simulink model "Q2"  (R2023a)
settings: Solver=VariableStepAuto  StartTime=0.0  StopTime=20  RelTol=1e-3
settings Model: Creator=DELL  LastModifiedBy=DELL

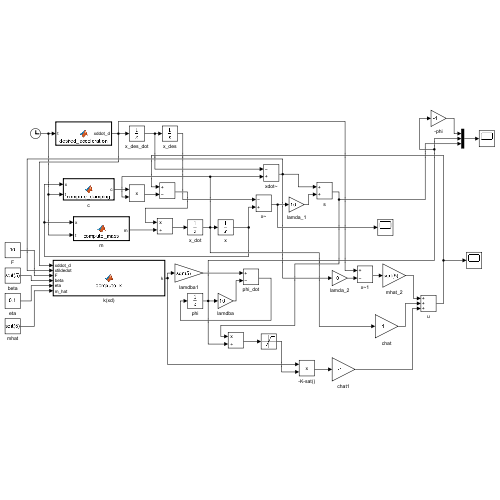
[thumbnail: Simulink's stored preview of the top-level diagram]
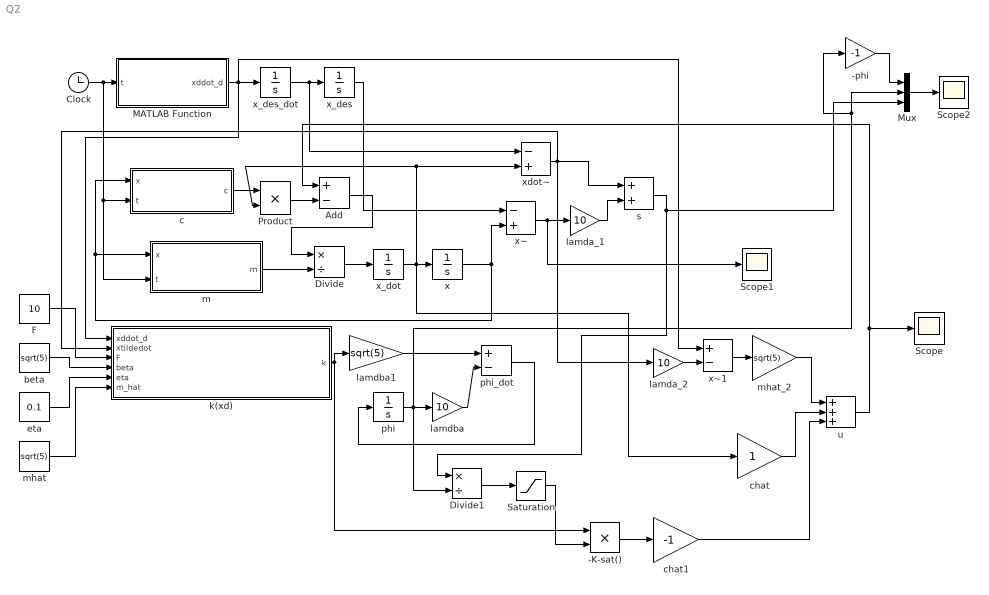
== system Q2 ==
  -K-sat() : Product  Inputs=**
  -phi : Gain  Gain=-1
  Add : Sum  Inputs=+-
  Clock : Clock
  Divide : Product  Inputs=*/
  Divide1 : Product  Inputs=*/
  F : Constant  Value=10
  MATLAB Function : MATLAB Function  TreatAsAtomicUnit=on
  Mux : Mux  Inputs=3
  Product : Product
  Saturation : Saturate  UpperLimit=1  LowerLimit=-1
  Scope : Scope
  Scope1 : Scope
  Scope2 : Scope
  beta : Constant  Value=sqrt(5)
  c : MATLAB Function  TreatAsAtomicUnit=on
  chat : Gain
  chat1 : Gain  Gain=-1
  eta : Constant  Value=0.1
  k(xd) : MATLAB Function  TreatAsAtomicUnit=on
  lamda_1 : Gain  Gain=10
  lamda_2 : Gain  Gain=10
  lamdba : Gain  Gain=10
  lamdba1 : Gain  Gain=sqrt(5)
  m : MATLAB Function  TreatAsAtomicUnit=on
  mhat : Constant  Value=sqrt(5)
  mhat_2 : Gain  Gain=sqrt(5)
  phi : Integrator  InitialCondition=0.01
  phi_dot : Sum  Inputs=+-
  s : Sum
  u : Sum  Inputs=+++
  x : Integrator
  x_des : Integrator
  x_des_dot : Integrator
  x_dot : Integrator
  xdot~ : Sum  Inputs=-+
  x~ : Sum  Inputs=-+
  x~1 : Sum  Inputs=+-
  wires:
  x_des_dot/1 -> xdot~/1, x_des/1
  Clock/1 -> c/2(t), m/2(t), MATLAB Function/1(t)
  MATLAB Function/1(xddot_d) -> x~1/1, k(xd)/1(xddot_d), x_des_dot/1
  m/1(m) -> Divide/2
  Divide/1 -> x_dot/1
  c/1(c) -> Product/1
  Product/1 -> Add/2
  Add/1 -> Divide/1
  x/1 -> m/1(x), c/1(x), x~/2
  x_des/1 -> x~/1
  x~/1 -> Scope1/1, lamda_1/1
  lamda_1/1 -> s/2
  xdot~/1 -> lamda_2/1, s/1, k(xd)/2(xtildedot)
  F/1 -> k(xd)/3(F)
  beta/1 -> k(xd)/4(beta)
  eta/1 -> k(xd)/5(eta)
  mhat/1 -> k(xd)/6(m_hat)
  phi/1 -> lamdba/1, Mux/2, -phi/1, Divide1/2
  lamdba/1 -> phi_dot/2
  x~1/1 -> mhat_2/1
  lamda_2/1 -> x~1/2
  x_dot/1 -> chat/1, x/1, xdot~/2, Product/2
  s/1 -> Mux/3, Divide1/1
  mhat_2/1 -> u/1
  chat/1 -> u/2
  u/1 -> Scope/1, Add/1
  Divide1/1 -> Saturation/1
  Saturation/1 -> -K-sat()/2
  phi_dot/1 -> phi/1
  -K-sat()/1 -> chat1/1
  Mux/1 -> Scope2/1
  -phi/1 -> Mux/1
  k(xd)/1(k) -> -K-sat()/1, lamdba1/1
  lamdba1/1 -> phi_dot/1
  chat1/1 -> u/3

== matlab function Q2/MATLAB Function ==
  data: t input; xddot_d output
function xddot_d = desired_acceleration(t)
    if t < 2
        xddot_d = 2;       % Acceleration phase (2 m/s²)
    elseif t >= 4 && t < 6
        xddot_d = -2;      % Deceleration phase (-2 m/s²)
    else
        xddot_d = 0;       % Constant velocity (4 m/s)
    end
end

== matlab function Q2/m ==
  data: x input; m output; t input
function m = compute_mass(x, t)
    m = 3 + 1.5 * sin(abs(x) * t);
end

== matlab function Q2/c ==
  data: x input; c output; t input
function c = compute_damping(x, t)
    c = 1.2 + 0.2 * sin(abs(x) * t);
end

== matlab function Q2/k(xd) ==
  data: xddot_d input; k output; xtildedot input; F input; beta input; eta input; m_hat input
function k = compute_k(xddot_d, xtildedot, F, beta, eta, m_hat)
    k = beta*(F + eta) +  (beta - 1) * abs(m_hat*xddot_d + 1 * xtildedot);
end
